simulink model "Project_1_final"  (R2023b)
settings: Solver=VariableStepAuto  StartTime=0.0  StopTime=10.0  RelTol=1e-3
values from neighbouring files (symbols this model uses):
  A = [1,100]    [Project1_Part2.m]    (also in Project_1_Final_Code.m = A_initial(A_index))
  b = b_initial(b_index)    [Project_1_Final_Code.m]
  frequency = 0    [Project_1_Final_Code.m]
  J = J_initial(J_index)    [Project_1_Final_Code.m]
  stiffness = [10, 100, 1000]    [Project_1_Final_Code.m]
  w_0 = w_0_initial(w_0_index)    [Project_1_Final_Code.m]
settings Model: Creator=rahma  LastModifiedBy=xavie

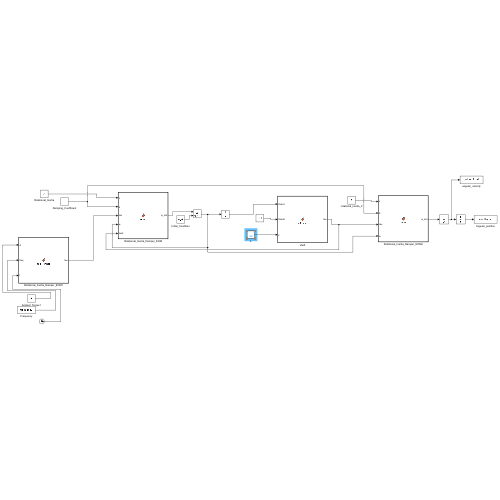
[thumbnail: Simulink's stored preview of the top-level diagram]
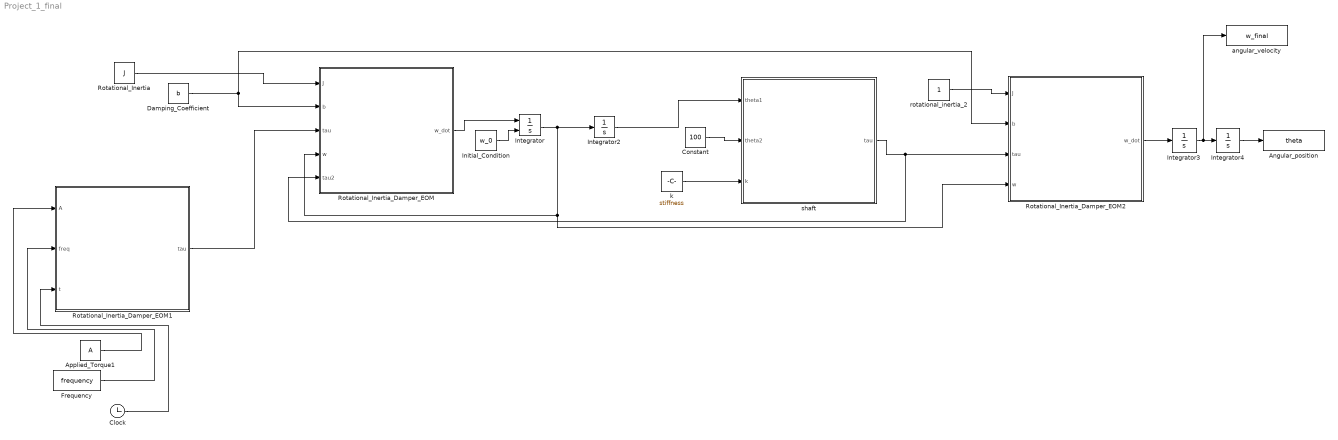
== system Project_1_final ==
  Angular_position : ToWorkspace  VariableName=theta  SaveFormat=Timeseries  SampleTime=-1
  Applied_Torque1 : Constant  Value=A
  Clock : Clock
  Constant : Constant  Value=100
  Damping_Coefficient : Constant  Value=b
  Frequency : Constant  Value=frequency
  Initial_Condition : Constant  Value=w_0
  Integrator : Integrator  InitialConditionSource=external
  Integrator2 : Integrator
  Integrator3 : Integrator
  Integrator4 : Integrator
  Rotational_Inertia : Constant  Value=J
  Rotational_Inertia_Damper_EOM : MATLAB Function  TreatAsAtomicUnit=on
  Rotational_Inertia_Damper_EOM1 : MATLAB Function  TreatAsAtomicUnit=on
  Rotational_Inertia_Damper_EOM2 : MATLAB Function  TreatAsAtomicUnit=on
  angular_velocity : ToWorkspace  VariableName=w_final  SaveFormat=Timeseries  SampleTime=-1
  k : Constant  Value=stiffness
  rotational_inertia_2 : Constant
  shaft : MATLAB Function  TreatAsAtomicUnit=on
  wires:
  Damping_Coefficient/1 -> Rotational_Inertia_Damper_EOM/2(b), Rotational_Inertia_Damper_EOM2/2(b)
  Integrator/1 -> Integrator2/1, Rotational_Inertia_Damper_EOM2/4(w), Rotational_Inertia_Damper_EOM/4(w)
  Rotational_Inertia/1 -> Rotational_Inertia_Damper_EOM/1(J)
  Rotational_Inertia_Damper_EOM/1(w_dot) -> Integrator/1
  Initial_Condition/1 -> Integrator/2
  shaft/1(tau) -> Rotational_Inertia_Damper_EOM/5(tau2), Rotational_Inertia_Damper_EOM2/3(tau)
  Integrator2/1 -> shaft/1(theta1)
  k/1 -> shaft/3(k)
  rotational_inertia_2/1 -> Rotational_Inertia_Damper_EOM2/1(J)
  Rotational_Inertia_Damper_EOM2/1(w_dot) -> Integrator3/1
  Integrator3/1 -> angular_velocity/1, Integrator4/1
  Integrator4/1 -> Angular_position/1
  Rotational_Inertia_Damper_EOM1/1(tau) -> Rotational_Inertia_Damper_EOM/3(tau)
  Frequency/1 -> Rotational_Inertia_Damper_EOM1/2(freq)
  Clock/1 -> Rotational_Inertia_Damper_EOM1/3(t)
  Applied_Torque1/1 -> Rotational_Inertia_Damper_EOM1/1(A)
  Constant/1 -> shaft/2(theta2)

== matlab function Project_1_final/Rotational_Inertia_Damper_EOM2 ==
  data: J input; w_dot output; b input; tau input; w input
function w_dot = eom(J, b, tau, w)
% Recall EOM: J*w_dot = tau_applied - tau_damped
tau_damped = b.*w;
% tau = A.*sin(freq.*t);
w_dot = (1/J)*(tau - tau_damped);
end

== matlab function Project_1_final/Rotational_Inertia_Damper_EOM ==
  data: J input; w_dot output; b input; tau input; w input; tau2 input
function w_dot = eom(J, b, tau, w, tau2)
% Recall EOM: J*w_dot = tau_applied - tau_damped
tau_damped = b.*w;
% tau = A.*sin(freq.*t);
w_dot = (1/J)*(tau - tau_damped);
end

== matlab function Project_1_final/shaft ==
  data: theta1 input; tau output; theta2 input; k input
function tau = stiffness(theta1,theta2,k)
% Recall EOM: J*w_dot = tau_applied - tau_damped
tau=k*(theta1-theta2);
% tau = A.*sin(freq.*t);
end

== matlab function Project_1_final/Rotational_Inertia_Damper_EOM1 ==
  data: A input; freq input; tau output; t input
function tau = app_torque(A, freq, t) % recieving values
if freq == 0 % since sine wave only happens if there is a frequency 
    tau = A; 
else 
    tau = A.*sin(freq.*t);
end
